simulink model "V2_TES_air"  (R2025b)
settings: Solver=VariableStepAuto  StartTime=0.0  StopTime=3600*9  RelTol=1e-3
model workspace (MAT data in the model file):
  COP = 3.9
  P1 = 1.04
  P2 = 1.91
  P3 = 1.91
  P4 = 1.05
  Q_Cond = 4.361
  Q_Evap = 3.471
  T1 = 12
  T2 = 37.72
  T3 = 29.61
  T4 = 7.9
  T_Enviroment_C = 27.5
  T_Room_int_C = 19.5
  h1 = 522.3
  h2 = 528.6
  h3 = 253.4
  h4 = 253.4
  m_dot = 0.014
libraries: fl_lib x25, nesl_utility x15, SimscapeFluids_lib x12
(part 2 of 2)

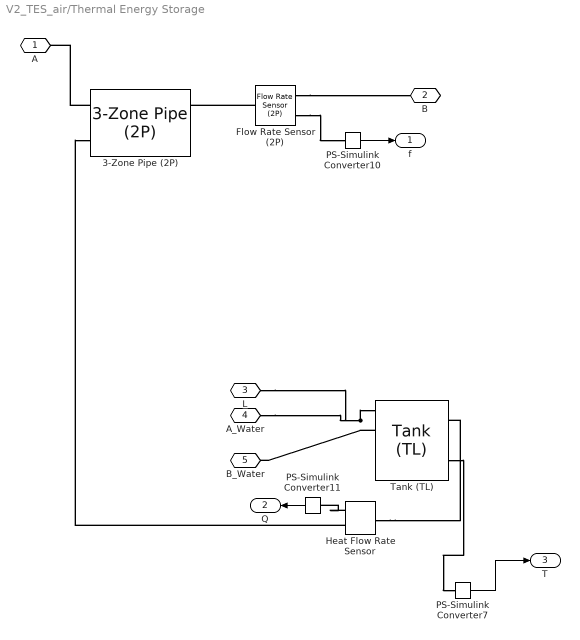
== system V2_TES_air/Thermal Energy Storage ==
  3-Zone Pipe (2P) : SimscapeFluids_lib/Two-Phase Fluid/Pipes & Fittings/3-Zone Pipe (2P)  length=L_Coil m  area=CrossDai_Area_tank m^2  Dh=Hydraulic_Daimeter m  elevation_gain=0 m  g=9.81 m/s^2  length_add=0.1 m  roughness=15e-6 m  Re_lam=2000  Re_tur=4000  shape_factor=64  hc_ext=h_Enviroment W/(K*m^2)  wall_thickness=Thinkness m  k_wall=Tube_k W/(K*m)  c_wall=Tube_Specific J/(K*kg)  rho_wall=Tube_Density kg/m^3  fin_ratio_ext=0  eta_fin_ext=0.6  fin_ratio_int=0  eta_fin_int=0.5  heat_coeff_spec=fluids.two_phase_fluid.pipes_fittings.enum.HeatCoeffSpec.GnielinskiCavalliniZecchin  colburn_coeff_liq=[.023, .8, .33]  colburn_coeff_mix=[.05, .8, .33]  colburn_coeff_vap=[.023, .8, .33]  Nu_lam=3.66  energy_spec=foundation.enum.energy_spec.temperature  p_init=P_int MPa  T_init=T_int degC  x_init=0.5  alpha_init=0.5  h_init=1500 kJ/kg  u_init=1500 kJ/kg
      settings: InternalSimscapePortConfiguration="{\"Bottom\":[],\"Left\":[{\"id\":\"A\",\"label\":\"A\",\"type\":\"foundation.two_phase_fluid.two_phase_fluid\"},{\"id\":\"H\",\"label\":\"H\",\"type\":\"foundation.thermal.thermal\"}],\"Right\":[{\"id\":\"B\",\"label\":\"B\",\"type\":\"foundation.two_phase_fluid.two_phase_fluid\"},{\"id\":\"Z\",\"label\":\"Z\",\"type\":\"output\"}],\"Top\":[]}"
  Flow Rate Sensor (2P) : fl_lib/Two-Phase Fluid/Sensors/Flow Rate Sensor (2P)  mass_flow_measure=true  volumetric_flow_measure=false  energy_flow_measure=false
      settings: InternalSimscapePortConfiguration="{\"Bottom\":[],\"Left\":[{\"id\":\"A\",\"label\":\"A\",\"type\":\"foundation.two_phase_fluid.two_phase_fluid\"}],\"Right\":[{\"id\":\"B\",\"label\":\"B\",\"type\":\"foundation.two_phase_fluid.two_phase_fluid\"},{\"id\":\"M\",\"label\":\"M\",\"type\":\"output\"}],\"Top\":[]}"
  Heat Flow Rate Sensor : fl_lib/Thermal/Thermal Sensors/Heat Flow Rate Sensor
  PS-Simulink Converter10 : nesl_utility/PS-Simulink Converter  PhysicalDomain=network_engine_domain  SubClassName=ps_output  LeftPortType=input  RightPortType=output  PseudoPeriodic=off  Frequencies=[]  VectorFormat=inherit  Unit=inherit  AffineConversion=off
  PS-Simulink Converter11 : nesl_utility/PS-Simulink Converter  PhysicalDomain=network_engine_domain  SubClassName=ps_output  LeftPortType=input  RightPortType=output  PseudoPeriodic=off  Frequencies=[]  VectorFormat=inherit  Unit=kW  AffineConversion=on
  PS-Simulink Converter7 : nesl_utility/PS-Simulink Converter  PhysicalDomain=network_engine_domain  SubClassName=ps_output  LeftPortType=input  RightPortType=output  PseudoPeriodic=off  Frequencies=[]  VectorFormat=inherit  Unit=degC  AffineConversion=on
  Tank (TL) : SimscapeFluids_lib/Thermal Liquid/Tanks & Accumulators/Tank (TL)  num_inlet=fluids.thermal_liquid.tanks_accumulators.enum.NumInlet.Two  pressure_spec=fluids.thermal_liquid.tanks_accumulators.enum.TankPressureSpec.Atmospheric  tank_pressure=0.101325 MPa  volume_spec=fluids.thermal_liquid.tanks_accumulators.enum.TankVolumeSpec.Constant  tank_area=Cross_area_Tank m^2  level_TLU=[0, 3, 5] m  volume_TLU=[0, 4, 6] m^3  inlet_height_A=0.1 m  inlet_area_A=0.01 m^2  inlet_heights_AB=[.1, LiquidMass/1000/Cross_area_Tank-0.1] m  inlet_areas_AB=[Port_Cross_area, Port_Cross_area] m^2  inlet_heights_ABC=[.1, .1, .1] m  inlet_areas_ABC=[.01, .01, .01] m^2  inlet_heights_ABCD=0.1 * ones(1, 4) m  inlet_areas_ABCD=0.01 * ones(1, 4) m^2  inlet_heights_ABCDE=0.1 * ones(1, 5) m  inlet_areas_ABCDE=0.01 * ones(1, 5) m^2  inlet_heights_ABCDEF=0.1 * ones(1, 6) m  inlet_areas_ABCDEF=0.01 * ones(1, 6) m^2  level_check=simscape.enum.assert.action.error  capacity_check=simscape.enum.assert.action.none  max_capacity=10 m^3  g=9.81 m/s^2  level_specify=on  level_priority=High  level=LiquidMass/1000/Cross_area_Tank m  level_nominal_specify=on  level_nominal_value=LiquidMass/1000/Cross_area_Tank  level_nominal_unit=m  volume_specify=off  volume_priority=None  volume=5 m^3  volume_nominal_specify=off  volume_nominal_value=1  volume_nominal_unit=m^3  mass_specify=on  mass_priority=None  mass=LiquidMass kg  mass_nominal_specify=off  mass_nominal_value=1  mass_nominal_unit=kg  T_I_specify=on  T_I_priority=High  T_I=273.15+T_int_tank K  T_I_nominal_specify=off  T_I_nominal_value=1  T_I_nominal_unit=K
      settings: InternalSimscapePortConfiguration="{\"Bottom\":[{\"id\":\"H\",\"label\":\"H\",\"type\":\"foundation.thermal.thermal\"},{\"id\":\"T_out\",\"label\":\"T\",\"type\":\"output\"}],\"Left\":[{\"id\":\"A\",\"label\":\"A\",\"type\":\"foundation.thermal_liquid.thermal_liquid\"},{\"id\":\"B\",\"label\":\"B\",\"type\":\"foundation.thermal_liquid.thermal_liquid\"}],\"Right\":[],\"Top\":[{\"id\":\"V_out\",\"label\":\"V\",\"type\":\"output\"},{\"id\":\"L_out\",\"label\":\"L\",\"type\":\"output\"}]}"
  A : PMIOPort  Side=Left
  B : PMIOPort  Port=2  Side=Left
  L : PMIOPort  Port=3  Side=Left
  A_Water : PMIOPort  Port=4  Side=Right
  B_Water : PMIOPort  Port=5  Side=Right
  f : Outport
  Q : Outport  Port=2
  T : Outport  Port=3
  wires:
  PS-Simulink Converter11/1 -> Q/1
  PS-Simulink Converter7/1 -> T/1
  PS-Simulink Converter10/1 -> f/1
  connections:
  Flow Rate Sensor (2P)/LConn1 -- 3-Zone Pipe (2P)/RConn1
  Heat Flow Rate Sensor/RConn1 -- PS-Simulink Converter11/LConn1
  Tank (TL)/LConn1 -- A_Water/RConn1 -- L/RConn1
  Heat Flow Rate Sensor/RConn2 -- 3-Zone Pipe (2P)/LConn2
  Tank (TL)/RConn2 -- PS-Simulink Converter7/LConn1
  Heat Flow Rate Sensor/LConn1 -- Tank (TL)/RConn1
  Flow Rate Sensor (2P)/RConn2 -- PS-Simulink Converter10/LConn1
  3-Zone Pipe (2P)/LConn1 -- A/RConn1
  Tank (TL)/LConn2 -- B_Water/RConn1
  Flow Rate Sensor (2P)/RConn1 -- B/RConn1
